simulink subsystem "Day1_Scenario_2"  (R2024a)
settings: Solver=VariableStepAuto  StartTime=0.0  StopTime=10.0  RelTol=1e-3
libraries: CarMaker4SL x2
settings Model: Creator=junhyung.cha  LastModifiedBy=junhyung.cha

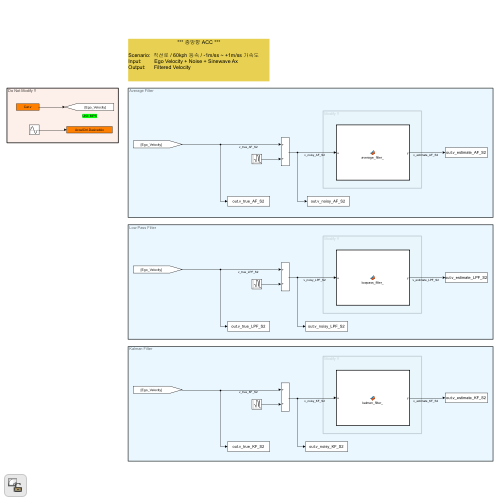
[thumbnail: Simulink's stored preview of the top-level diagram]
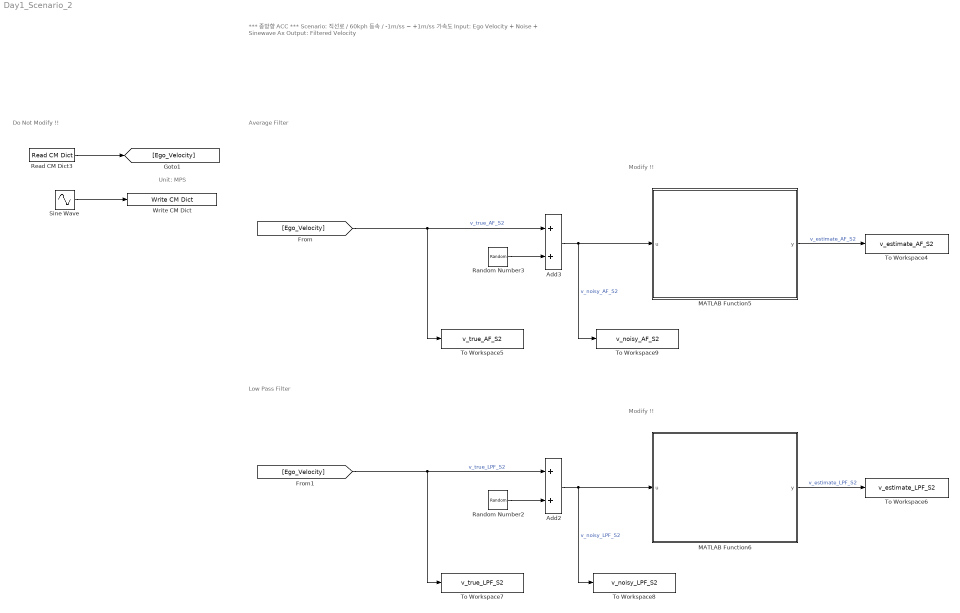
== system Day1_Scenario_2 ==
  note: Do Not Modify !!
  note: Low Pass Filter
  note: Average Filter
  note: Modify !!
  note: Modify !!
  note: *** 종방향 ACC ***
      |
      | Scenario: 직선로 / 60kph 등속 / -1m/ss ~ +1m/ss 가속도
      | Input: Ego Velocity + Noise + Sinewave Ax
      | Output: Filtered Velocity
  note: Unit: MPS
  Add2 : Sum
  Add3 : Sum
  MATLAB Function5 : MATLAB Function  TreatAsAtomicUnit=on
  MATLAB Function6 : MATLAB Function  TreatAsAtomicUnit=on
  Random Number2 : RandomNumber
  Random Number3 : RandomNumber
  Read CM Dict3 : CarMaker4SL/Read CM Dict  xname=Car.v  xsync=off  xstime=Inherited
  Sine Wave : Sin
  To Workspace4 : ToWorkspace  VariableName=v_estimate_AF_S2  SaveFormat=Timeseries  SampleTime=-1
  To Workspace5 : ToWorkspace  VariableName=v_true_AF_S2  SaveFormat=Timeseries  SampleTime=-1
  To Workspace6 : ToWorkspace  VariableName=v_estimate_LPF_S2  SaveFormat=Timeseries  SampleTime=-1
  To Workspace7 : ToWorkspace  VariableName=v_true_LPF_S2  SaveFormat=Timeseries  SampleTime=-1
  To Workspace8 : ToWorkspace  VariableName=v_noisy_LPF_S2  SaveFormat=Timeseries  SampleTime=-1
  To Workspace9 : ToWorkspace  VariableName=v_noisy_AF_S2  SaveFormat=Timeseries  SampleTime=-1
  Write CM Dict : CarMaker4SL/Write CM Dict  xname=AccelCtrl.DesiredAx  xsync=off
  wires:
  Sine Wave/1 -> Write CM Dict/1
  Random Number3/1 -> Add3/2
  Add3/1 -> To Workspace9/1, MATLAB Function5/1(u)  "v_noisy_AF_S2"
  Add2/1 -> To Workspace8/1, MATLAB Function6/1(u)  "v_noisy_LPF_S2"
  [Ego_Velocity] -> Add2/1, To Workspace7/1  "v_true_LPF_S2"
  MATLAB Function6/1(y) -> To Workspace6/1  "v_estimate_LPF_S2"
  Random Number2/1 -> Add2/2
  MATLAB Function5/1(y) -> To Workspace4/1  "v_estimate_AF_S2"
  [Ego_Velocity] -> Add3/1, To Workspace5/1  "v_true_AF_S2"
  Read CM Dict3/1 -> [Ego_Velocity]

== matlab function Day1_Scenario_2/MATLAB Function6 ==
  settings: updateMethod=DISCRETE  sampleTime=0.05
  data: u input; y output
function y = lowpass_filter_(u)
    y = 0;
end

== matlab function Day1_Scenario_2/MATLAB Function5 ==
  settings: updateMethod=DISCRETE  sampleTime=0.05
  data: u input; y output
function y = average_filter_(u)
    y = 0;
end
